simulink model "model2_control_LgV"  (R2025b)
settings: Solver=ode45  StartTime=0.0  StopTime=10  MaxStep=0.00012566370614359171  RelTol=1e-7  AbsTol=1e-9
values from neighbouring files (symbols this model uses):
  p = [g; L; zeta; A; f]    [kapitza_controle.m]    (also in parameters_kapitza_model2.m)
  pc = [c1; c2; alpha_ctrl]    [kapitza_controle.m]
  x0 = [150*pi/180; 0]    [kapitza_controle.m]    (also in parameters_kapitza_model2.m = [45*pi/180; 0])
settings Model: Creator=rafae  LastModifiedBy=rafae
settings SolverCC: AutoScaleAbsTol=off

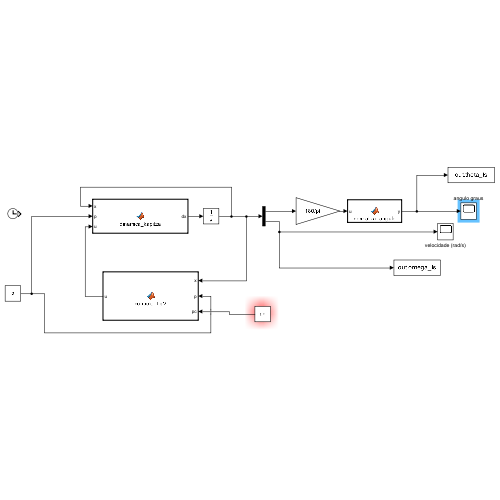
[thumbnail: Simulink's stored preview of the top-level diagram]
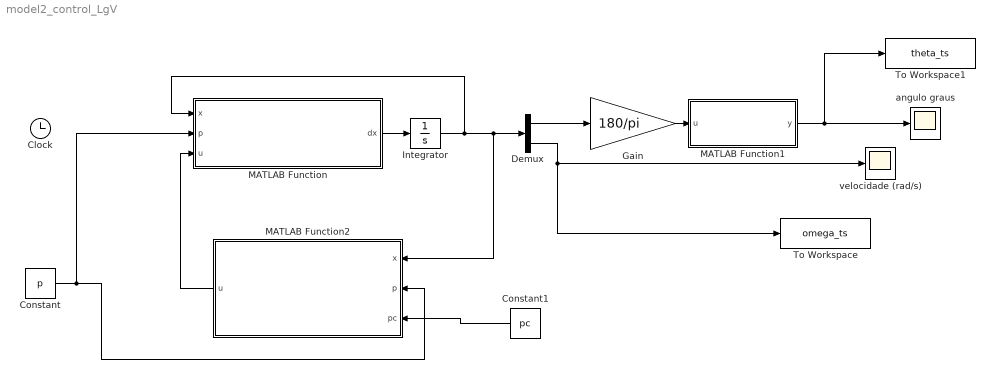
== system model2_control_LgV ==
  Clock : Clock
  Constant : Constant  Value=p
  Constant1 : Constant  Value=pc
  Demux : Demux  Outputs=2
  Gain : Gain  Gain=180/pi
  Integrator : Integrator  InitialCondition=x0
  MATLAB Function : MATLAB Function  TreatAsAtomicUnit=on
  MATLAB Function1 : MATLAB Function  TreatAsAtomicUnit=on
  MATLAB Function2 : MATLAB Function  TreatAsAtomicUnit=on
  To Workspace : ToWorkspace  VariableName=omega_ts  SaveFormat=Timeseries  SampleTime=-1
  To Workspace1 : ToWorkspace  VariableName=theta_ts  SaveFormat=Timeseries  SampleTime=-1
  angulo graus : Scope
      settings: ActiveDisplayYMinimum=-150.27555928856486  ActiveDisplayYMaximum=2.4800335970836436
  velocidade (rad/s) : Scope
      settings: ActiveDisplayYMinimum=-1  ActiveDisplayYMaximum=1
  wires:
  Constant/1 -> MATLAB Function/2(p), MATLAB Function2/2(p)
  MATLAB Function/1(dx) -> Integrator/1
  Integrator/1 -> MATLAB Function/1(x), MATLAB Function2/1(x), Demux/1
  Demux/2 -> velocidade (rad/s)/1, To Workspace/1
  Gain/1 -> MATLAB Function1/1(u)
  Demux/1 -> Gain/1
  MATLAB Function1/1(y) -> To Workspace1/1, angulo graus/1
  Constant1/1 -> MATLAB Function2/3(pc)
  MATLAB Function2/1(u) -> MATLAB Function/3(u)

== matlab function model2_control_LgV/MATLAB Function1 ==
  data: u input; y output
function y = normaliza_angulo(u)
    y = mod(u + 180, 360) - 180;
end

== matlab function model2_control_LgV/MATLAB Function ==
  data: x input; p input; dx output; u input
function dx = dinamica_kapitza(x, p, u)%#codegen

g = p(1);
L = p(2);
zeta = p(3);


theta = x(1);
velocidade = x(2);

wn = sqrt(g/L);

dx = zeros(2,1);
dx(1) = velocidade;

dx(2) = -2*zeta*wn*velocidade ...
        + (g/L-u/L)*sin(theta);
end

== matlab function model2_control_LgV/MATLAB Function2 ==
  data: x input; u output; p input; pc input
function u = controle_LgV(x, p, pc)
%#codegen

L = p(2);

c2 = pc(2);
alpha_ctrl = pc(3);

theta = x(1);
velocidade = x(2);

u = (c2*alpha_ctrl/L)*sin(theta) ...
       *(c2*velocidade + sin(theta));

end
